simulink model "vibracion_auto"  (Simulink 7.5)
settings: Solver=ode45  StartTime=0.0  StopTime=20  RelTol=1e-3
settings Model: Creator=JuanC  LastModifiedBy=JuanC

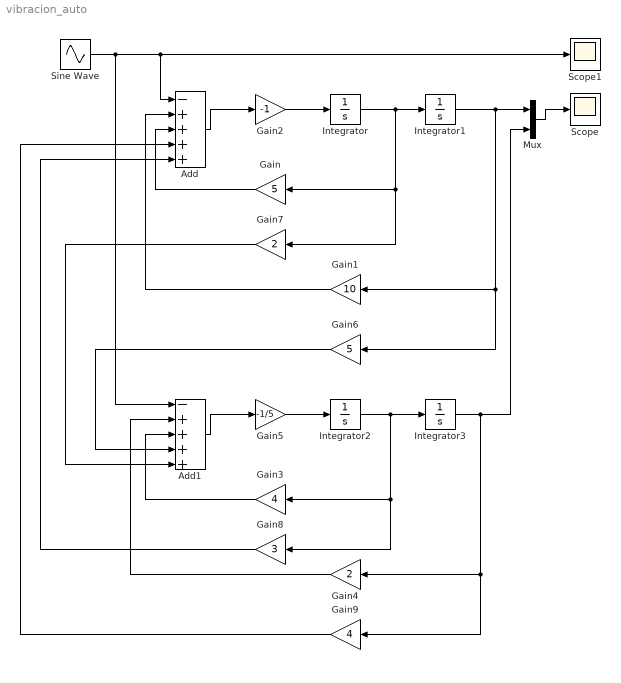
== system vibracion_auto ==
  Add : Sum  Inputs=-++++  OutDataType=fixdt(1, 16)  OutScaling=2^-10
  Add1 : Sum  Inputs=-++++  OutDataType=fixdt(1, 16)  OutScaling=2^-10
  Gain : Gain  Gain=5  ParameterDataType=fixdt(1, 16)  ParameterScaling=2^0  OutDataType=fixdt(1, 16)  OutScaling=2^0
  Gain1 : Gain  Gain=10  ParameterDataType=fixdt(1, 16)  ParameterScaling=2^0  OutDataType=fixdt(1, 16)  OutScaling=2^0
  Gain2 : Gain  Gain=-1  ParameterDataType=fixdt(1, 16)  ParameterScaling=2^0  OutDataType=fixdt(1, 16)  OutScaling=2^0
  Gain3 : Gain  Gain=4  ParameterDataType=fixdt(1, 16)  ParameterScaling=2^0  OutDataType=fixdt(1, 16)  OutScaling=2^0
  Gain4 : Gain  Gain=2  ParameterDataType=fixdt(1, 16)  ParameterScaling=2^0  OutDataType=fixdt(1, 16)  OutScaling=2^0
  Gain5 : Gain  Gain=-1/5  ParameterDataType=fixdt(1, 16)  ParameterScaling=2^0  OutDataType=fixdt(1, 16)  OutScaling=2^0
  Gain6 : Gain  Gain=5  ParameterDataType=fixdt(1, 16)  ParameterScaling=2^0  OutDataType=fixdt(1, 16)  OutScaling=2^0
  Gain7 : Gain  Gain=2  ParameterDataType=fixdt(1, 16)  ParameterScaling=2^0  OutDataType=fixdt(1, 16)  OutScaling=2^0
  Gain8 : Gain  Gain=3  ParameterDataType=fixdt(1, 16)  ParameterScaling=2^0  OutDataType=fixdt(1, 16)  OutScaling=2^0
  Gain9 : Gain  Gain=4  ParameterDataType=fixdt(1, 16)  ParameterScaling=2^0  OutDataType=fixdt(1, 16)  OutScaling=2^0
  Integrator{,1..3} (4 alike) : Integrator
  Mux : Mux  Inputs=2
  Scope : Scope
  Scope1 : Scope
  Sine Wave : Sin  Amplitude=1  Bias=0  Frequency=1  Phase=0  Samples=10  SampleTime=0  Offset=0
  wires:
  Integrator/1 -> Integrator1/1, Gain/1, Gain7/1
  Integrator1/1 -> Gain1/1, Gain6/1, Mux/1
  Gain2/1 -> Integrator/1
  Sine Wave/1 -> Add/1, Scope1/1, Add1/1
  Add/1 -> Gain2/1
  Gain/1 -> Add/3
  Gain1/1 -> Add/2
  Integrator2/1 -> Integrator3/1, Gain3/1, Gain8/1
  Integrator3/1 -> Gain4/1, Gain9/1, Mux/2
  Gain5/1 -> Integrator2/1
  Add1/1 -> Gain5/1
  Gain3/1 -> Add1/3
  Gain4/1 -> Add1/2
  Gain8/1 -> Add/5
  Gain9/1 -> Add/4
  Gain6/1 -> Add1/4
  Gain7/1 -> Add1/5
  Mux/1 -> Scope/1
